simulink subsystem "SRP_torque"  (R2022b)
settings: Solver=VariableStepAuto  StartTime=0.0  StopTime=10.0  RelTol=1e-3
undefined symbols (not defined in the file or in its folder): environment, sat
libraries: matrix_library x7, vrlib x1
settings Model: Creator=Nicolò  LastModifiedBy=Nicolò

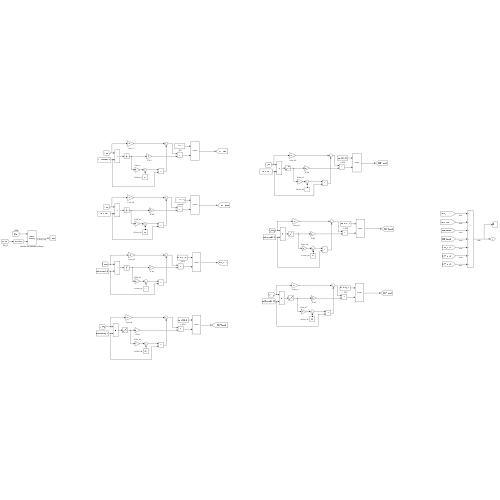
[thumbnail: Simulink's stored preview of the top-level diagram]
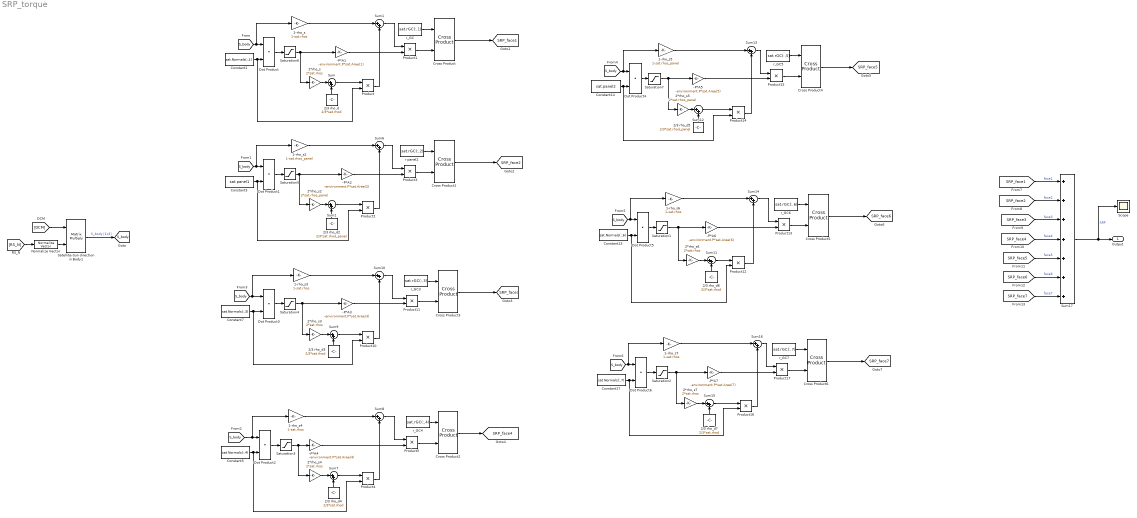
== system SRP_torque ==
  -P*A1 : Gain  Gain=-environment.P*sat.Aree(1)
  -P*A2 : Gain  Gain=-environment.P*sat.Aree(2)
  -P*A3 : Gain  Gain=-environment.P*sat.Aree(3)
  -P*A4 : Gain  Gain=-environment.P*sat.Aree(4)
  -P*A5 : Gain  Gain=-environment.P*sat.Aree(5)
  -P*A6 : Gain  Gain=-environment.P*sat.Aree(6)
  -P*A7 : Gain  Gain=-environment.P*sat.Aree(7)
  1-rho_s{,3..4,6..7} (5 alike) : Gain  Gain=1-sat.rhos
  1-rho_s2 : Gain  Gain=1-sat.rhos_panel
  1-rho_s5 : Gain  Gain=1-sat.rhos_panel
  2*rho_s{,3..4,6..7} (5 alike) : Gain  Gain=2*sat.rhos
  2*rho_s2 : Gain  Gain=2*sat.rhos_panel
  2*rho_s5 : Gain  Gain=2*sat.rhos_panel
  2/3 rho_d{,3..4,6..7} (5 alike) : Constant  Value=2/3*sat.rhod
  2/3 rho_d2 : Constant  Value=2/3*sat.rhod_panel
  2/3 rho_d5 : Constant  Value=2/3*sat.rhod_panel
  Constant1 : Constant  Value=sat.Normals(:,1)
  Constant13 : Constant  Value=sat.Normals(:,6)
  Constant14 : Constant  Value=sat.panel2
  Constant17 : Constant  Value=sat.Normals(:,7)
  Constant3 : Constant  Value=sat.panel1
  Constant5 : Constant  Value=sat.Normals(:,4)
  Constant7 : Constant  Value=sat.Normals(:,3)
  Cross Product{,1..6} (7 alike) : matrix_library/Cross Product
  Dot Product{,1..6} (7 alike) : DotProduct  OutDataTypeStr=Inherit: Inherit via internal rule
  Normalize Vector : vrlib/Utilities/Normalize Vector  maxzero=0
  Product{,1..5,10..17} (14 alike) : Product
  Satellite-Sun direction in Body1 : Product  Multiplication=Matrix(*)
  Saturation{1..7} (7 alike) : Saturate  UpperLimit=1  LowerLimit=0
  Scope : Scope
  Sum{,1..2,6..16} (14 alike) : Sum  Inputs=|++
  Sum17 : Sum  Inputs=+++++++
  r panel2 : Constant  Value=sat.rGC(:,2)
  r_GC : Constant  Value=sat.rGC(:,1)
  r_GC3 : Constant  Value=sat.rGC(:,3)
  r_GC4 : Constant  Value=sat.rGC(:,4)
  r_GC5 : Constant  Value=sat.rGC(:,5)
  r_GC6 : Constant  Value=sat.rGC(:,6)
  r_GC7 : Constant  Value=sat.rGC(:,7)
  Output : Outport
  tag scope: SRP_face1=global, SRP_face2=global, SRP_face3=global, SRP_face4=global, SRP_face5=global, SRP_face6=global, SRP_face7=global, S_body=global
  wires:
  Sum7/1 -> Product4/1
  [S_body] -> 1-rho_s4/1, Dot Product2/1
  Constant3/1 -> Dot Product1/2, Product2/2
  Product3/1 -> Cross Product1/2
  1-rho_s2/1 -> Sum6/1
  -P*A1/1 -> Product1/2
  Sum1/1 -> Product1/1
  Product4/1 -> Sum8/2
  Sum/1 -> Product/1
  1-rho_s3/1 -> Sum10/1
  2/3 rho_d/1 -> Sum/2
  [S_body] -> 1-rho_s/1, Dot Product/1
  Constant1/1 -> Product/2, Dot Product/2
  Sum9/1 -> Product10/1
  -P*A3/1 -> Product11/2
  Product11/1 -> Cross Product3/2
  r_GC3/1 -> Cross Product3/1
  r_GC5/1 -> Cross Product4/1
  Sum8/1 -> Product5/1
  Product14/1 -> Sum13/2
  -P*A5/1 -> Product15/2
  Sum12/1 -> Product14/1
  1-rho_s5/1 -> Sum13/1
  Product/1 -> Sum1/2
  2/3 rho_d5/1 -> Sum12/2
  Cross Product1/1 -> [SRP_face2]
  r_GC4/1 -> Cross Product2/1
  r_GC/1 -> Cross Product/1
  Satellite-Sun direction in Body1/1 -> [S_body]  "S_body [1x3]"
  2*rho_s/1 -> Sum/1
  Product5/1 -> Cross Product2/2
  Dot Product4/1 -> Saturation7/1
  -P*A4/1 -> Product5/2
  [S_body] -> 1-rho_s5/1, Dot Product4/1
  Product10/1 -> Sum10/2
  -P*A2/1 -> Product3/2
  Dot Product1/1 -> Saturation5/1
  2*rho_s5/1 -> Sum12/1
  1-rho_s4/1 -> Sum8/1
  Sum16/1 -> Product17/1
  Sum17/1 -> Output/1, Scope/1  "SRP"
  [SRP_face3] -> Sum17/3  "face3"
  2/3 rho_d2/1 -> Sum2/2
  Dot Product2/1 -> Saturation3/1
  [SRP_face1] -> Sum17/1  "face1"
  -P*A7/1 -> Product17/2
  Cross Product6/1 -> [SRP_face7]
  [SRP_face4] -> Sum17/4  "face4"
  [SRP_face7] -> Sum17/7  "face7"
  Constant5/1 -> Product4/2, Dot Product2/2
  2/3 rho_d3/1 -> Sum9/2
  Cross Product/1 -> [SRP_face1]
  [SRP_face5] -> Sum17/5  "face5"
  [SRP_face2] -> Sum17/2  "face2"
  Sum2/1 -> Product2/1
  Dot Product3/1 -> Saturation4/1
  1-rho_s7/1 -> Sum16/1
  r_GC7/1 -> Cross Product6/1
  Product16/1 -> Sum16/2
  Cross Product2/1 -> [SRP_face4]
  r_GC6/1 -> Cross Product5/1
  Dot Product6/1 -> Saturation2/1
  Dot Product/1 -> Saturation6/1
  2*rho_s7/1 -> Sum15/1
  1-rho_s/1 -> Sum1/1
  2/3 rho_d7/1 -> Sum15/2
  Constant13/1 -> Dot Product5/2, Product12/2
  Sum11/1 -> Product12/1
  2*rho_s4/1 -> Sum7/1
  Product12/1 -> Sum14/2
  Product13/1 -> Cross Product5/2
  [S_body] -> 1-rho_s7/1, Dot Product6/1
  r panel2/1 -> Cross Product1/1
  Sum10/1 -> Product11/1
  Product2/1 -> Sum6/2
  [S_body] -> Dot Product1/1, 1-rho_s2/1
  Product15/1 -> Cross Product4/2
  1-rho_s6/1 -> Sum14/1
  Sum6/1 -> Product3/1
  [SRP_face6] -> Sum17/6  "face6"
  [S_body] -> Dot Product5/1, 1-rho_s6/1
  Product17/1 -> Cross Product6/2
  Product1/1 -> Cross Product/2
  Constant7/1 -> Dot Product3/2, Product10/2
  Constant14/1 -> Product14/2, Dot Product4/2
  [S_body] -> Dot Product3/1, 1-rho_s3/1
  Cross Product3/1 -> [SRP_face3]
  2/3 rho_d4/1 -> Sum7/2
  2*rho_s3/1 -> Sum9/1
  Dot Product5/1 -> Saturation1/1
  2*rho_s6/1 -> Sum11/1
  2*rho_s2/1 -> Sum2/1
  2/3 rho_d6/1 -> Sum11/2
  Sum13/1 -> Product15/1
  Cross Product5/1 -> [SRP_face6]
  -P*A6/1 -> Product13/2
  Constant17/1 -> Product16/2, Dot Product6/2
  Sum14/1 -> Product13/1
  Sum15/1 -> Product16/1
  [DCM] -> Satellite-Sun direction in Body1/1
  [RS_N] -> Normalize Vector/1
  Normalize Vector/1 -> Satellite-Sun direction in Body1/2
  Cross Product4/1 -> [SRP_face5]
  Saturation7/1 -> -P*A5/1, 2*rho_s5/1
  Saturation1/1 -> 2*rho_s6/1, -P*A6/1
  Saturation2/1 -> -P*A7/1, 2*rho_s7/1
  Saturation3/1 -> -P*A4/1, 2*rho_s4/1
  Saturation4/1 -> 2*rho_s3/1, -P*A3/1
  Saturation5/1 -> 2*rho_s2/1, -P*A2/1
  Saturation6/1 -> 2*rho_s/1, -P*A1/1
